simulink library "sim_operations"  (R2016a)
settings: Solver=ode45  StartTime=0.0  StopTime=10.0  RelTol=1e-3
libraries: Math_Lib x3
settings Model: Creator=sanny.omar  LastModifiedBy=Sanny
settings DataIOCC: LimitDataPoints=on  SaveFormat=Array
settings DebuggingCC: SolverPrmCheckMsg=warning
settings HardwareCC: ProdBitPerPointer=32  ProdLargestAtomicFloat=None  ProdIntDivRoundTo=Undefined  ProdEndianess=Unspecified  ProdWordSize=32  ProdHWDeviceType=32-bit Generic
settings ModelReferenceCC: PropagateSignalLabelsOutOfModel=off
settings ConfigComp: CovModelRefEnable=Off  CovSFcnEnable=off

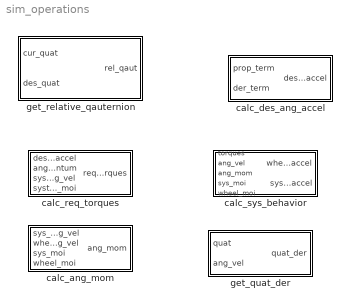
== system sim_operations ==
  calc_ang_mom : Subsystem
  calc_des_ang_accel : Subsystem
  calc_req_torques : Subsystem
  calc_sys_behavior : Subsystem
  get_quat_der : Subsystem
  get_relative_qauternion : Subsystem

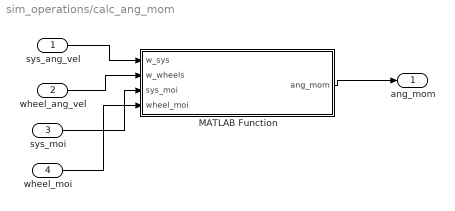
== system sim_operations/calc_ang_mom ==
  sys_ang_vel : Inport
  wheel_ang_vel : Inport  Port=2
  sys_moi : Inport  Port=3
  wheel_moi : Inport  Port=4
  MATLAB Function : MATLAB Function  TreatAsAtomicUnit=on
  ang_mom : Outport
  wires:
  sys_ang_vel/1 -> MATLAB Function/1(w_sys)
  wheel_ang_vel/1 -> MATLAB Function/2(w_wheels)
  MATLAB Function/1(ang_mom) -> ang_mom/1
  sys_moi/1 -> MATLAB Function/3(sys_moi)
  wheel_moi/1 -> MATLAB Function/4(wheel_moi)

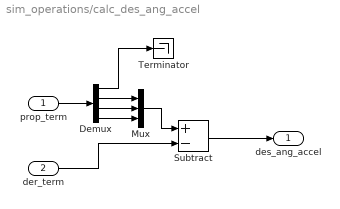
== system sim_operations/calc_des_ang_accel ==
  prop_term : Inport
  der_term : Inport  Port=2
  Demux : Demux
  Mux : Mux  Inputs=3
  Subtract : Sum  Inputs=+-
  Terminator : Terminator
  des_ang_accel : Outport
  wires:
  prop_term/1 -> Demux/1
  der_term/1 -> Subtract/2
  Subtract/1 -> des_ang_accel/1
  Demux/2 -> Mux/1
  Demux/3 -> Mux/2
  Demux/4 -> Mux/3
  Mux/1 -> Subtract/1
  Demux/1 -> Terminator/1

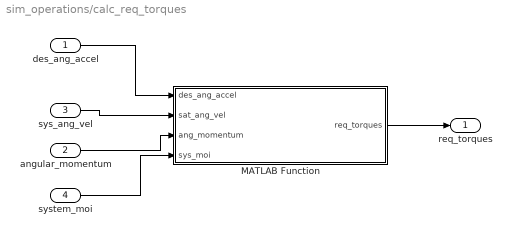
== system sim_operations/calc_req_torques ==
  des_ang_accel : Inport
  angular_momentum : Inport  Port=2
  sys_ang_vel : Inport  Port=3
  system_moi : Inport  Port=4
  MATLAB Function : MATLAB Function  TreatAsAtomicUnit=on
  req_torques : Outport
  wires:
  des_ang_accel/1 -> MATLAB Function/1(des_ang_accel)
  angular_momentum/1 -> MATLAB Function/3(ang_momentum)
  MATLAB Function/1(req_torques) -> req_torques/1
  sys_ang_vel/1 -> MATLAB Function/2(sat_ang_vel)
  system_moi/1 -> MATLAB Function/4(sys_moi)

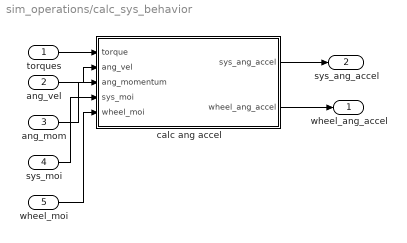
== system sim_operations/calc_sys_behavior ==
  torques : Inport
  ang_vel : Inport  Port=2
  ang_mom : Inport  Port=3
  sys_moi : Inport  Port=4
  wheel_moi : Inport  Port=5
  calc ang accel : MATLAB Function  TreatAsAtomicUnit=on
  wheel_ang_accel : Outport  PortDimensions=3
  sys_ang_accel : Outport  Port=2  PortDimensions=3
  wires:
  calc ang accel/2(wheel_ang_accel) -> wheel_ang_accel/1
  calc ang accel/1(sys_ang_accel) -> sys_ang_accel/1
  torques/1 -> calc ang accel/1(torque)
  ang_vel/1 -> calc ang accel/2(ang_vel)
  ang_mom/1 -> calc ang accel/3(ang_momentum)
  sys_moi/1 -> calc ang accel/4(sys_moi)
  wheel_moi/1 -> calc ang accel/5(wheel_moi)

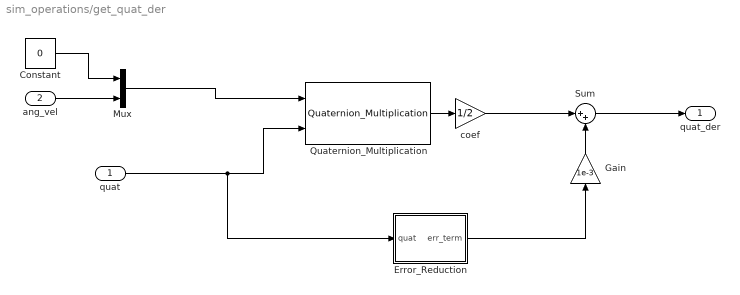
== system sim_operations/get_quat_der ==
  quat : Inport  PortDimensions=4
  ang_vel : Inport  Port=2  PortDimensions=3
  Constant : Constant  Value=0
  Error_Reduction : MATLAB Function  TreatAsAtomicUnit=on
  Gain : Gain  Gain=1e-3
  Mux : Mux  Inputs=2
  Quaternion_Multiplication : Math_Lib/Quaternion_Multiplication  Description=Multiplies two quaternions
  Sum : Sum  Inputs=|++
  coef : Gain  Gain=1/2
  quat_der : Outport
  wires:
  Quaternion_Multiplication/1 -> coef/1
  quat/1 -> Error_Reduction/1(quat), Quaternion_Multiplication/2
  Constant/1 -> Mux/1
  ang_vel/1 -> Mux/2
  Mux/1 -> Quaternion_Multiplication/1
  coef/1 -> Sum/1
  Error_Reduction/1(err_term) -> Gain/1
  Sum/1 -> quat_der/1
  Gain/1 -> Sum/2

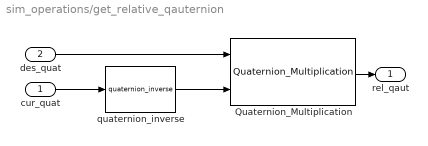
== system sim_operations/get_relative_qauternion ==
  cur_quat : Inport  PortDimensions=4
  des_quat : Inport  Port=2  PortDimensions=4
  Quaternion_Multiplication : Math_Lib/Quaternion_Multiplication
  quaternion_inverse : Math_Lib/quaternion_inverse
  rel_qaut : Outport
  wires:
  cur_quat/1 -> quaternion_inverse/1
  Quaternion_Multiplication/1 -> rel_qaut/1
  des_quat/1 -> Quaternion_Multiplication/1
  quaternion_inverse/1 -> Quaternion_Multiplication/2

== matlab function sim_operations/calc_req_torques/MATLAB Function ==
  data: des_ang_accel input; req_torques output; sat_ang_vel input; ang_momentum input; sys_moi input
% This function calculates the torques required to acheive a given satellite 
% angular acceleration. These 'required torques' can be acieved by applying a
% torque directly to the body or by accelerating a reaction wheel such that
% the wheel accelerates opposite the direction of the desired body torque
% vector
function req_torques = calc_torques(des_ang_accel, sat_ang_vel, ang_momentum, sys_moi)
    req_torques = sys_moi*des_ang_accel - cross(ang_momentum, sat_ang_vel);
end

== matlab function sim_operations/get_quat_der/Error_Reduction ==
  data: quat input; err_term output
function err_term = reduce_error(quat)
    error = 1-norm(quat);
    err_term = quat*error;
end

== matlab function sim_operations/calc_sys_behavior/calc ang accel ==
  data: torque input; sys_ang_accel output; ang_vel input; ang_momentum input; wheel_ang_accel output; sys_moi input; wheel_moi input
% This function calculates the angular acceleration vector of a body based
% on the body's moment of inertia matrix, angular momentum vector,
% angular momentum derivative, and angular velocity vector, and a 
% vector of applied torques
function [sys_ang_accel, wheel_ang_accel] = calc_ang_accel(torque, ang_vel, ang_momentum, sys_moi, wheel_moi)
    % Calculations based on equation dH/dt = H x w + T
    ang_mom_der = cross(ang_momentum, ang_vel) + torque;
    sys_ang_accel = (inv(sys_moi))*ang_mom_der;
    wheel_ang_accel = -torque/wheel_moi;
end

== matlab function sim_operations/calc_ang_mom/MATLAB Function ==
  data: w_sys input; ang_mom output; w_wheels input; sys_moi input; wheel_moi input
function ang_mom = get_ang_mom(w_sys, w_wheels, sys_moi, wheel_moi)
    % This function gets the total angular momentum of the system
    ang_mom = sys_moi*w_sys + wheel_moi*w_wheels;
